simulink model "quadrator_model_v2"  (R2022b)
settings: Solver=FixedStepAuto  StartTime=0.0  StopTime=50  FixedStep=0.001  MaxStep=0.001  RelTol=1e-3
values from neighbouring files (symbols this model uses):
  l = readmatrix("RampTest_2023-06-05_114458")    [pwm2thrust_lut.m]
undefined symbols (not defined in the file or in its folder): manu
libraries: slpidlib x12, matrix_library x8, aerolibutil x7, sharedtransform x4, sharedutil x4, simulink_extras x3, shared6dof x1, aerolibasang x1, dspmathops x1
(part 1 of 2)
settings Model: Creator=ata  LastModifiedBy=ata
settings SolverCC: ZeroCrossAlgorithm=Adaptive
settings DataIOCC: Refine=4

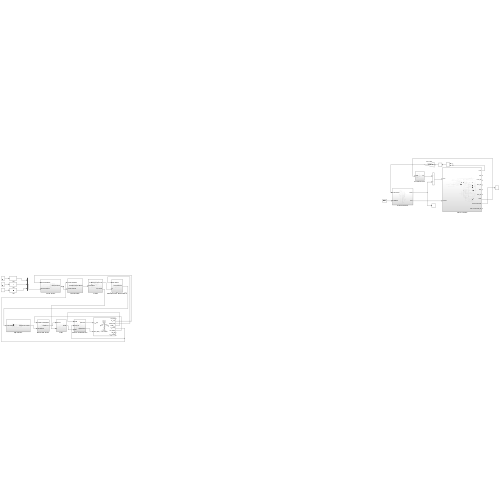
[thumbnail: Simulink's stored preview of the top-level diagram]
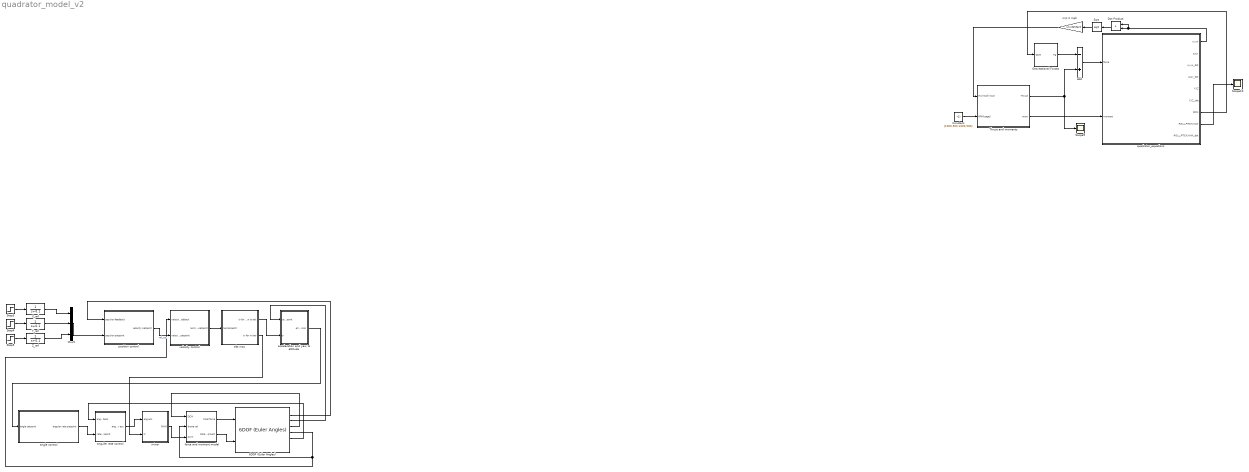
== system quadrator_model_v2 ==
  6DOF (Euler Angles) : shared6dof/6DOF (Euler Angles)  units=Metric (MKS)  mtype=Fixed  rep=Euler Angles  xme_0=[0 0 0]  Vm_0=[0.01 0.01 0.01]  eul_0=[0 0 0]  pm_0=[0 0 0]  mass_0=7.5  mass_e=0.5  mass_f=2.0  inertia=[0.3, 0,0 ; 0,0.3,0 ; 0,0, 0.2434]  inertia_e=eye(3)  inertia_f=2*eye(3)  k_quat=1.0  vre_flag=on  abi_flag=off  aMode=0  xme_statename=''  Vm_statename=''  eul_statename=''  quat_statename=''  pm_statename=''  mass_statename=''
  Add : Sum  Inputs=-+
  Constant : Constant  Value=[1000,500,1000,500]
  Dot Product : DotProduct  OutDataTypeStr=Inherit: Inherit via internal rule
  Gravitational Forces : Subsystem
  Mux5 : Mux  Inputs=3
  Scope10 : Scope
  Scope9 : Scope
  Sqrt : Sqrt
  Step3 : Step  After=2  SampleTime=0
  Step4 : Step  After=3  SampleTime=0
  Step5 : Step  After=-2  SampleTime=0
  Thrust and moments : Subsystem
  X_ref : TransferFcn  Denominator=[1 0.1]
  Y_ref : TransferFcn  Denominator=[1 0.1]
  Z_ref : TransferFcn  Denominator=[1 0.1]
  acceleration and yaw to attitude : Subsystem
  angle control : Subsystem
  anguler rate control : Subsystem
  force and moment model : Subsystem
  m/s 2 mph : Gain  Gain=1/2.23693629
  mixer : Subsystem
  position control : Subsystem
  quadrotor_equations : Subsystem
  tiltt max : Subsystem
  velocity control : Subsystem
  wires:
  quadrotor_equations/7(DCM) -> Gravitational Forces/1(DCM)
  Add/1 -> quadrotor_equations/1(force)
  quadrotor_equations/1(u,v,w) -> Dot Product/1, Dot Product/2
  Dot Product/1 -> Sqrt/1
  Constant/1 -> Thrust and moments/2(RPM(page))
  Sqrt/1 -> m/s 2 mph/1
  m/s 2 mph/1 -> Thrust and moments/1(Hız(mph)(row))
  Gravitational Forces/1(Fg) -> Add/1
  Thrust and moments/1(Thrust) -> Scope9/1, Add/2
  Thrust and moments/2(mom) -> quadrotor_equations/2(moment)
  quadrotor_equations/8(ROLL,PITCH,YAW) -> Scope10/1
  6DOF (Euler Angles)/2 -> position control/1(position feedback)
  6DOF (Euler Angles)/6 -> anguler rate control/1(angular rate feedback)
  6DOF (Euler Angles)/5 -> velocity control/1(velocity feedback), force and moment model/2(drone vel)
  6DOF (Euler Angles)/3 -> acceleration and yaw to attitude/1(yaw setpoint)
  position control/1(velocity setpoint) -> velocity control/2(velocity setpoint)  "vel_sp"
  velocity control/1(normalized thrust setpoint) -> tiltt max/1(nomalised tr)
  tiltt max/1(tr for Acc and Yaw to att) -> acceleration and yaw to attitude/2(tr)
  acceleration and yaw to attitude/1(error quaternion) -> angle control/1(angle setpoint)
  angle control/1(angular rate setpoint) -> anguler rate control/2(rate setpoint)
  anguler rate control/1(angular acc) -> mixer/1(ang acc)
  tiltt max/2(tr for mixer) -> mixer/2(tr)
  6DOF (Euler Angles)/4 -> force and moment model/1(DCM)
  mixer/1(PWM) -> force and moment model/3(pwm)
  force and moment model/1(total force) -> 6DOF (Euler Angles)/1
  force and moment model/2(total moment) -> 6DOF (Euler Angles)/2
  Mux5/1 -> position control/2(position setpoint)
  Y_ref/1 -> Mux5/2
  Step5/1 -> Z_ref/1
  Step3/1 -> X_ref/1
  X_ref/1 -> Mux5/1
  Z_ref/1 -> Mux5/3
  Step4/1 -> Y_ref/1

== system quadrator_model_v2/Gravitational Forces ==
  DCM : Inport
  G : Constant  Value=9.81
  Matrix Multiply : Product  Multiplication=Matrix(*)
  Product : Product
  Vector Concatenate : Concatenate  ConcatenateDimension=2
  mass : Constant  Value=7.5
  mass2 : Constant  Value=zeros(2,1)  VectorParams1D=off
  Fg : Outport
  wires:
  Matrix Multiply/1 -> Fg/1
  mass/1 -> Product/2
  mass2/1 -> Vector Concatenate/1
  G/1 -> Product/1
  Product/1 -> Vector Concatenate/2
  Vector Concatenate/1 -> Matrix Multiply/2
  DCM/1 -> Matrix Multiply/1

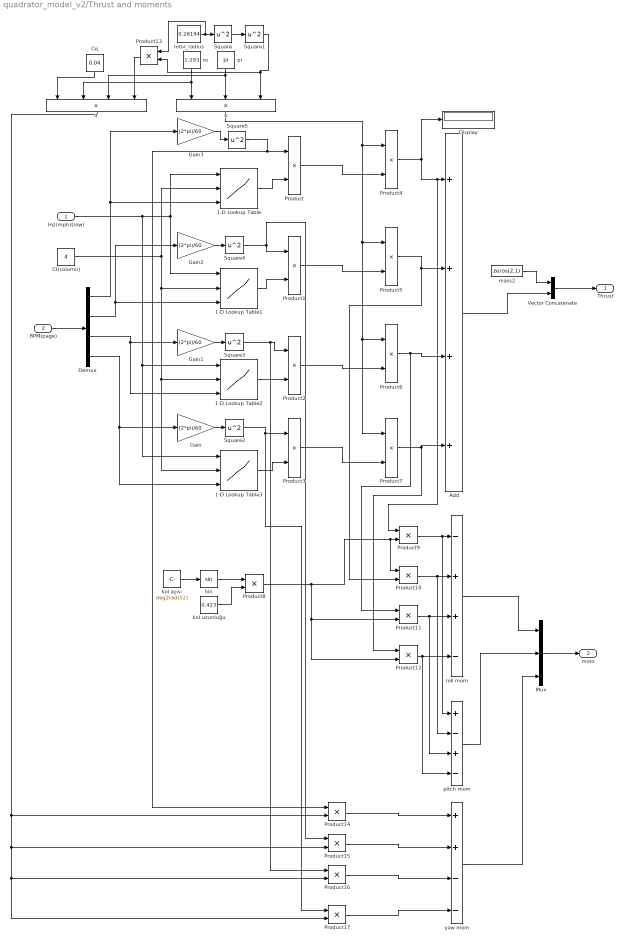
== system quadrator_model_v2/Thrust and moments ==
  Hız(mph)(row) : Inport
  RPM(page) : Inport  Port=2
  1-D Lookup Table : Lookup_n-D  NumberOfTableDimensions=3  BreakpointsForDimension1=manu(:,1)  BreakpointsForDimension2=(1:1:15)  BreakpointsForDimension3=(1000:1000:11000)  Table=manu  ExtrapMethod=Clip  UseLastTableValue=on  InternalRulePriority=Speed  RndMeth=Simplest
      settings: InputPortMap=u0,u1,u2
  1-D Lookup Table1 : Lookup_n-D  NumberOfTableDimensions=3  BreakpointsForDimension1=manu(:,1)  BreakpointsForDimension2=(1:1:15)  BreakpointsForDimension3=(1000:1000:11000)  Table=manu  ExtrapMethod=Clip  UseLastTableValue=on  InternalRulePriority=Speed  RndMeth=Simplest
      settings: InputPortMap=u0,u1,u2
  1-D Lookup Table2 : Lookup_n-D  NumberOfTableDimensions=3  BreakpointsForDimension1=manu(:,1)  BreakpointsForDimension2=(1:1:15)  BreakpointsForDimension3=(1000:1000:11000)  Table=manu  ExtrapMethod=Clip  UseLastTableValue=on  InternalRulePriority=Speed  RndMeth=Simplest
      settings: InputPortMap=u0,u1,u2
  1-D Lookup Table3 : Lookup_n-D  NumberOfTableDimensions=3  BreakpointsForDimension1=manu(:,1)  BreakpointsForDimension2=(1:1:15)  BreakpointsForDimension3=(1000:1000:11000)  Table=manu  ExtrapMethod=Clip  InternalRulePriority=Speed  RndMeth=Simplest
      settings: InputPortMap=u0,u1,u2
  Add : Sum  Inputs=++++
  Cq : Constant  Value=0.04
  Ct(column) : Constant  Value=4
  Demux : Demux
  Display : Display
  Gain{,1..3} (4 alike) : Gain  Gain=(2*pi)/60
  Mux : Mux  Inputs=3
  Product{,1..17} (18 alike) : Product
  Sin : Trigonometry
  Square{,1..5} (6 alike) : Math  Operator=square
  Vector Concatenate : Concatenate  ConcatenateDimension=2
  b : Product  Inputs=3
  d : Product  Inputs=4
  kol açısı : Constant  Value=deg2rad(52)
  kol uzunluğu : Constant  Value=0.423
  mass2 : Constant  Value=zeros(2,1)  VectorParams1D=off
  pi : Constant  Value=pi
  pitch mom : Sum  Inputs=+-+-
  ro : Constant  Value=1.293
  roll mom : Sum  Inputs=-++-
  rotor_radius : Constant  Value=0.28194
  yaw mom : Sum  Inputs=++--
  Thrust : Outport
  mom : Outport  Port=2
  wires:
  Product4/1 -> Display/1, Product9/1, Add/1
  Product7/1 -> Product12/1, Add/4
  Product2/1 -> Product6/2
  Square5/1 -> Product14/1, Product/1
  Product/1 -> Product4/2
  Gain2/1 -> Square4/1
  Product3/1 -> Product7/2
  Gain1/1 -> Square3/1
  Square3/1 -> Product2/1, Product16/1
  Square4/1 -> Product1/1, Product15/1
  1-D Lookup Table2/1 -> Product2/2
  Square2/1 -> Product17/1, Product3/1
  RPM(page)/1 -> Demux/1
  Gain3/1 -> Square5/1
  Product5/1 -> Product10/2, Add/2
  1-D Lookup Table/1 -> Product/2
  1-D Lookup Table3/1 -> Product3/2
  Gain/1 -> Square2/1
  1-D Lookup Table1/1 -> Product1/2
  pi/1 -> b/2, d/3
  Square1/1 -> Product13/2, b/3
  Product6/1 -> Product11/1, Add/3
  Demux/4 -> 1-D Lookup Table3/3, Gain/1
  ro/1 -> d/2, b/1
  Square/1 -> Square1/1
  Demux/1 -> Gain3/1, 1-D Lookup Table/3
  Demux/3 -> 1-D Lookup Table2/3, Gain1/1
  b/1 -> Product4/1, Product7/1, Product6/1, Product5/1
  Hız(mph)(row)/1 -> 1-D Lookup Table/1, 1-D Lookup Table1/1, 1-D Lookup Table3/1, 1-D Lookup Table2/1
  Demux/2 -> Gain2/1, 1-D Lookup Table1/3
  Ct(column)/1 -> 1-D Lookup Table/2, 1-D Lookup Table2/2, 1-D Lookup Table3/2, 1-D Lookup Table1/2
  rotor_radius/1 -> Product13/1, Square/1
  Product1/1 -> Product5/2
  mass2/1 -> Vector Concatenate/1
  Vector Concatenate/1 -> Thrust/1
  Add/1 -> Vector Concatenate/2
  kol açısı/1 -> Sin/1
  Sin/1 -> Product8/1
  kol uzunluğu/1 -> Product8/2
  Product8/1 -> Product12/2, Product11/2, Product10/1, Product9/2
  Product9/1 -> pitch mom/1, roll mom/1
  Product10/1 -> pitch mom/2, roll mom/2
  Product11/1 -> pitch mom/3, roll mom/3
  Product12/1 -> roll mom/4, pitch mom/4
  roll mom/1 -> Mux/1
  pitch mom/1 -> Mux/2
  Mux/1 -> mom/1
  Cq/1 -> d/1
  Product13/1 -> d/4
  yaw mom/1 -> Mux/3
  d/1 -> Product17/2, Product16/2, Product15/2, Product14/2
  Product14/1 -> yaw mom/1
  Product15/1 -> yaw mom/2
  Product16/1 -> yaw mom/3
  Product17/1 -> yaw mom/4

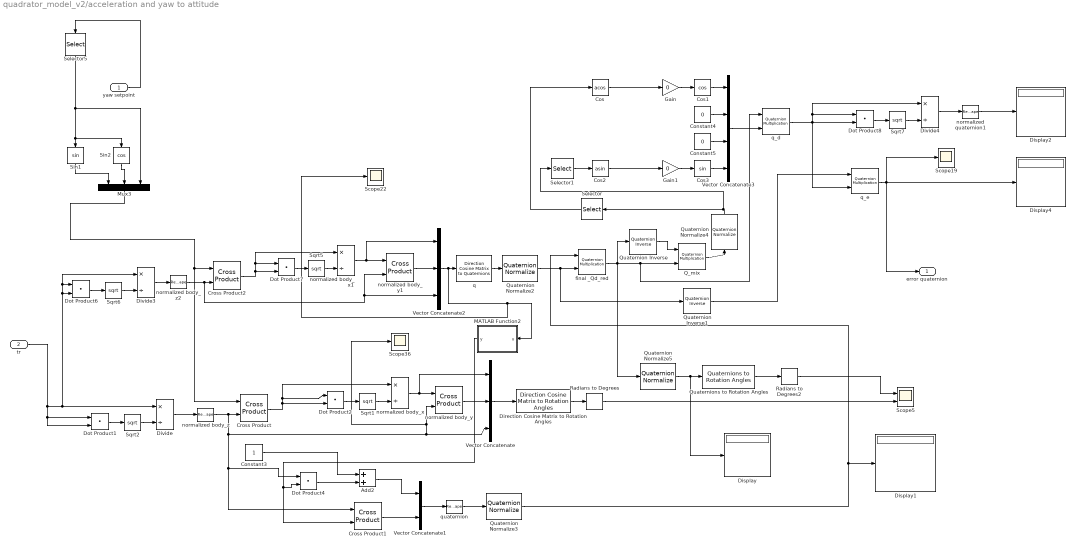
== system quadrator_model_v2/acceleration and yaw to attitude ==
  yaw setpoint : Inport
  tr : Inport  Port=2
  Add2 : Sum
  Constant3 : Constant
  Constant4 : Constant  Value=0
  Constant5 : Constant  Value=0
  Cos : Trigonometry  Operator=acos
  Cos1 : Trigonometry  Operator=cos
  Cos2 : Trigonometry  Operator=asin
  Cos3 : Trigonometry
  Cross Product : matrix_library/Cross Product
  Cross Product1 : matrix_library/Cross Product
  Cross Product2 : matrix_library/Cross Product
  Direction Cosine Matrix to Rotation Angles : sharedtransform/Direction Cosine Matrix to Rotation Angles  rotationOrder=ZYX  aMode=aMode  action=None  tolerance=eps(2)
      settings: LibrarySourceBlock=|
      | aerolibtransform2/Direction Cosine Matrix
      | to Rotation Angles
  Display{,1..2,4} (4 alike) : Display
  Divide : Product  Inputs=*/
  Divide3 : Product  Inputs=*/
  Divide4 : Product  Inputs=*/
  Dot Product{1..2,4,6..8} (6 alike) : DotProduct  OutDataTypeStr=Inherit: Inherit via internal rule
  Gain : Gain  Gain=0
  Gain1 : Gain  Gain=0
  MATLAB Function2 : MATLAB Function  TreatAsAtomicUnit=on
  Mux3 : Mux  Inputs=3
  Q_mix : aerolibutil/Quaternion Multiplication
  Quaternion Inverse : aerolibutil/Quaternion Inverse
  Quaternion Inverse1 : aerolibutil/Quaternion Inverse
  Quaternion Normalize{2..5} (4 alike) : sharedutil/Quaternion Normalize  aMode=aMode
  Quaternions to Rotation Angles : sharedtransform/Quaternions to Rotation Angles  rotationOrder=ZYX  aMode=aMode
  Radians to Degrees : simulink_extras/Transformations/Radians to Degrees
  Radians to Degrees2 : simulink_extras/Transformations/Radians to Degrees
  Scope19 : Scope
  Scope22 : Scope
  Scope36 : Scope
  Scope5 : Scope  NumInputPorts=2
  Selector : Selector  InputPortWidth=4  IndexOptions=Index vector (dialog)  Indices=[1]  OutputSizes=1
  Selector1 : Selector  InputPortWidth=4  IndexOptions=Index vector (dialog)  Indices=[4]  OutputSizes=1
  Selector5 : Selector  InputPortWidth=3  IndexOptions=Index vector (dialog)  Indices=[ 3]  OutputSizes=1
  Sin1 : Trigonometry
  Sin2 : Trigonometry  Operator=cos
  Sqrt{1..2,5..7} (5 alike) : Sqrt
  Vector Concatenate : Concatenate  NumInputs=3  Mode=Multidimensional array  ConcatenateDimension=2
  Vector Concatenate1 : Concatenate  ConcatenateDimension=2
  Vector Concatenate2 : Concatenate  NumInputs=3  Mode=Multidimensional array  ConcatenateDimension=2
  Vector Concatenate3 : Concatenate  NumInputs=4  Mode=Multidimensional array  ConcatenateDimension=2
  final _Qd_red : aerolibutil/Quaternion Multiplication
  normalized body_x : Product  Inputs=*/
  normalized body_x1 : Product  Inputs=*/
  normalized body_y : matrix_library/Cross Product
  normalized body_y1 : matrix_library/Cross Product
  normalized body_z : Reshape  OutputDimensionality=Column vector (2-D)
  normalized body_z2 : Reshape  OutputDimensionality=Column vector (2-D)
  normalized quaternion1 : Reshape  OutputDimensionality=Column vector (2-D)
  q : sharedtransform/Direction Cosine Matrix  to Quaternions  aMode=0  action=None  tolerance=eps(2)
      settings: LibrarySourceBlock=|
      | aerolibtransform2/Direction Cosine Matrix
      | to Quaternions
  q_d : aerolibutil/Quaternion Multiplication
  q_e : aerolibutil/Quaternion Multiplication
  quaternion : Reshape  OutputDimensionality=Row vector (2-D)
  error quaternion : Outport
  wires:
  yaw setpoint/1 -> Selector5/1
  Cos/1 -> Gain/1
  q/1 -> Quaternion Normalize2/1
  Divide4/1 -> normalized quaternion1/1
  Cos3/1 -> Vector Concatenate3/4
  Selector1/1 -> Cos2/1
  Add2/1 -> Vector Concatenate1/1
  Quaternion Inverse/1 -> Q_mix/1
  Cross Product1/1 -> Vector Concatenate1/2
  Vector Concatenate/1 -> Direction Cosine Matrix to Rotation Angles/1
  Sqrt1/1 -> normalized body_x/2
  Dot Product7/1 -> Sqrt5/1
  Sin1/1 -> Mux3/1
  Radians to Degrees/1 -> Scope5/2
  q_d/1 -> Divide4/1, Dot Product8/1, Dot Product8/2, q_e/2
  Quaternion Normalize3/1 -> Display1/1, final _Qd_red/1
  final _Qd_red/1 -> Quaternion Normalize5/1, Quaternion Inverse/1, q_d/1, Q_mix/2
  Radians to Degrees2/1 -> Scope5/1
  Sqrt2/1 -> Divide/2
  normalized body_x1/1 -> normalized body_y1/1, Vector Concatenate2/1
  Sqrt6/1 -> Divide3/2
  Quaternion Normalize5/1 -> Display/1, Quaternions to Rotation Angles/1
  Sqrt5/1 -> normalized body_x1/2
  Cos1/1 -> Vector Concatenate3/1
  Constant5/1 -> Vector Concatenate3/3
  Gain/1 -> Cos1/1
  Cos2/1 -> Gain1/1
  Divide/1 -> normalized body_z/1
  Quaternion Normalize4/1 -> Selector1/1, Selector/1
  Selector/1 -> Cos/1
  Gain1/1 -> Cos3/1
  normalized body_z/1 -> Cross Product1/1, Dot Product4/1, Scope36/1, normalized body_y/2, Vector Concatenate/3, Cross Product/2
  Dot Product1/1 -> Sqrt2/1
  Quaternions to Rotation Angles/1 -> Radians to Degrees2/1
  Quaternion Inverse1/1 -> q_e/1
  Dot Product2/1 -> Sqrt1/1
  Sin2/1 -> Mux3/2
  Cross Product/1 -> normalized body_x/1, Dot Product2/1, Dot Product2/2
  normalized body_x/1 -> Vector Concatenate/1, normalized body_y/1
  Quaternion Normalize2/1 -> final _Qd_red/2, Quaternion Inverse1/1
  Vector Concatenate1/1 -> quaternion/1
  Vector Concatenate3/1 -> q_d/2
  Direction Cosine Matrix to Rotation Angles/1 -> Radians to Degrees/1
  normalized body_z2/1 -> Cross Product2/2, Vector Concatenate2/3, normalized body_y1/2
  Constant4/1 -> Vector Concatenate3/2
  tr/1 -> Divide/1, Dot Product6/2, Divide3/1, Dot Product6/1, Dot Product1/2, Dot Product1/1
  quaternion/1 -> Quaternion Normalize3/1
  Selector5/1 -> Mux3/3, Sin2/1, Sin1/1
  Dot Product8/1 -> Sqrt7/1
  Sqrt7/1 -> Divide4/2
  q_e/1 -> error quaternion/1, Scope19/1, Display4/1
  Dot Product6/1 -> Sqrt6/1
  Dot Product4/1 -> Add2/2
  normalized body_y/1 -> Vector Concatenate/2
  Divide3/1 -> normalized body_z2/1
  normalized quaternion1/1 -> Display2/1
  Q_mix/1 -> Quaternion Normalize4/1
  Mux3/1 -> Cross Product2/1, Cross Product/1
  normalized body_y1/1 -> Vector Concatenate2/2
  MATLAB Function2/1(y) -> Cross Product1/2, Dot Product4/2
  Vector Concatenate2/1 -> q/1, Scope22/1, MATLAB Function2/1(u)
  Constant3/1 -> Add2/1
  Cross Product2/1 -> normalized body_x1/1, Dot Product7/1, Dot Product7/2

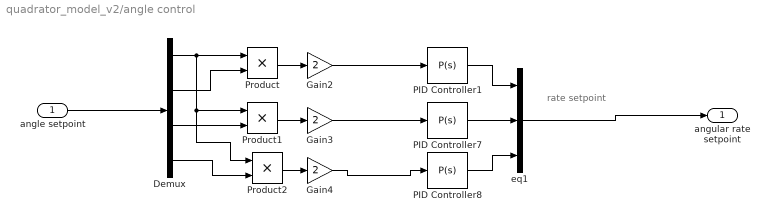
== system quadrator_model_v2/angle control ==
  note: rate setpoint
  angle setpoint : Inport
  Demux : Demux
  Gain2 : Gain  Gain=2
  Gain3 : Gain  Gain=2
  Gain4 : Gain  Gain=2
  PID Controller1 : slpidlib/PID Controller  Controller=P  Form=Parallel  TimeDomain=Continuous-time  UseExternalTs=off  SampleTime=-1  IntegratorMethod=Forward Euler  FilterMethod=Forward Euler  ControllerParametersSource=internal  P=20  I=9.5219837376893e-06  UseKiTs=off  D=-1.0490403925014e-05  N=1.72044274974478  UseFilter=on  TunerSelectOption=Transfer Function Based (PID Tuner App)  InitialConditionSource=internal  InitialConditionForIntegrator=0  InitialConditionForFilter=0  DifferentiatorICPrevScaledInput=0  ExternalReset=none  TrackingMode=off  Kt=1  LimitOutput=off  SatLimitsSource=internal  UpperSaturationLimit=inf  LowerSaturationLimit=-inf  LinearizeAsGain=on  AntiWindupMode=none  Kb=1  LimitIntegrator=off  UpperIntegratorSaturationLimit=inf  LowerIntegratorSaturationLimit=-inf  POutMin=[]  POutMax=[]  IOutMin=[]  IOutMax=[]  DOutMin=[]  DOutMax=[]  NOutMin=[]  NOutMax=[]  SumOutMin=[]  SumOutMax=[]  SaturationOutMin=[]  SaturationOutMax=[]  PParamMin=[]  PParamMax=[]  IParamMin=[]  IParamMax=[]  DParamMin=[]  DParamMax=[]  NParamMin=[]  NParamMax=[]  KbParamMin=[]  KbParamMax=[]  KtParamMin=[]  KtParamMax=[]  KbOutMin=[]  KbOutMax=[]  KtOutMin=[]  KtOutMax=[]  IntegratorOutMin=[]  IntegratorOutMax=[]  FilterOutMin=[]  FilterOutMax=[]  SumI1OutMin=[]  SumI1OutMax=[]  SumI2OutMin=[]  SumI2OutMax=[]  SumI3OutMin=[]  SumI3OutMax=[]  SumI4OutMin=[]  SumI4OutMax=[]  SumDOutMin=[]  SumDOutMax=[]  DifferentiatorOutMin=[]  DifferentiatorOutMax=[]  FilterDiffOutCoefMin=[]  FilterDiffOutCoefMax=[]  ReciprocalOutMin=[]  ReciprocalOutMax=[]  SumDenOutMin=[]  SumDenOutMax=[]  SumNumOutMin=[]  SumNumOutMax=[]  DivideOutMin=[]  DivideOutMax=[]  UdiffTsProdOutMin=[]  UdiffTsProdOutMax=[]  NTsProdOutMin=[]  NTsProdOutMax=[]  UintegralTsProdOutMin=[]  UintegralTsProdOutMax=[]  UngainTsProdOutMin=[]  UngainTsProdOutMax=[]  ClampingZeroOutDataTypeStr=Inherit: Inherit via back propagation  ClampingZeroOutMin=[]  ClampingZeroOutMax=[]  FilterDenConstantOutDataTypeStr=Inherit: Inherit via back propagation  FilterDenConstantOutMin=[]  FilterDenConstantOutMax=[]  PCopyOutDataTypeStr=Inherit: Inherit via back propagation  PCopyOutMin=[]  PCopyOutMax=[]  NCopyOutDataTypeStr=Inherit: Inherit via back propagation  NCopyOutMin=[]  NCopyOutMax=[]  IntegratorContinuousStateAttributes=''  IntegratorStateMustResolveToSignalObject=off  IntegratorRTWStateStorageClass=Auto  FilterContinuousStateAttributes=''  FilterStateMustResolveToSignalObject=off  FilterRTWStateStorageClass=Auto  ParallelPVariant=InternalParameters  IdealPVariant=Disabled  IVariant=Disabled  DVariant=Disabled  IntegratorVariant=Disabled  SatVariant=Disabled  AWVariant=Disabled  PCopyVariant=Disabled  TRVariant=Disabled  FdbkBlocksVariant=Forward  IdealPFdbkVariant=Disabled  SatFdbkVariant=Disabled  DerivativeFilterVariant=Disabled  NVariant=Disabled  NCopyVariant=Disabled_SignalSpec  FilterICVariant=Disabled  IntegratorICVariant=Disabled  ExternalResetVariant=Disabled  TRSumVariant=Passthrough  SumFdbkVariant=Disabled  SumVariant=Passthrough_P  TsampFilterVariant=InternalTs  TsampNgainVariant=Passthrough  TsampIntegralVariant=Disabled_SignalSpec  ExternalSaturationOutDataTypeStr=Inherit: Same as second input
  PID Controller7 : slpidlib/PID Controller  Controller=P  Form=Parallel  TimeDomain=Continuous-time  UseExternalTs=off  SampleTime=-1  IntegratorMethod=Forward Euler  FilterMethod=Forward Euler  ControllerParametersSource=internal  P=9.5  I=-6.49908455563329e-05  UseKiTs=off  D=-0.683044885728483  N=43.2582215401561  UseFilter=on  TunerSelectOption=Transfer Function Based (PID Tuner App)  InitialConditionSource=internal  InitialConditionForIntegrator=0  InitialConditionForFilter=0  DifferentiatorICPrevScaledInput=0  ExternalReset=none  TrackingMode=off  Kt=1  LimitOutput=off  SatLimitsSource=internal  UpperSaturationLimit=inf  LowerSaturationLimit=-inf  LinearizeAsGain=on  AntiWindupMode=none  Kb=1  LimitIntegrator=off  UpperIntegratorSaturationLimit=inf  LowerIntegratorSaturationLimit=-inf  POutMin=[]  POutMax=[]  IOutMin=[]  IOutMax=[]  DOutMin=[]  DOutMax=[]  NOutMin=[]  NOutMax=[]  SumOutMin=[]  SumOutMax=[]  SaturationOutMin=[]  SaturationOutMax=[]  PParamMin=[]  PParamMax=[]  IParamMin=[]  IParamMax=[]  DParamMin=[]  DParamMax=[]  NParamMin=[]  NParamMax=[]  KbParamMin=[]  KbParamMax=[]  KtParamMin=[]  KtParamMax=[]  KbOutMin=[]  KbOutMax=[]  KtOutMin=[]  KtOutMax=[]  IntegratorOutMin=[]  IntegratorOutMax=[]  FilterOutMin=[]  FilterOutMax=[]  SumI1OutMin=[]  SumI1OutMax=[]  SumI2OutMin=[]  SumI2OutMax=[]  SumI3OutMin=[]  SumI3OutMax=[]  SumI4OutMin=[]  SumI4OutMax=[]  SumDOutMin=[]  SumDOutMax=[]  DifferentiatorOutMin=[]  DifferentiatorOutMax=[]  FilterDiffOutCoefMin=[]  FilterDiffOutCoefMax=[]  ReciprocalOutMin=[]  ReciprocalOutMax=[]  SumDenOutMin=[]  SumDenOutMax=[]  SumNumOutMin=[]  SumNumOutMax=[]  DivideOutMin=[]  DivideOutMax=[]  UdiffTsProdOutMin=[]  UdiffTsProdOutMax=[]  NTsProdOutMin=[]  NTsProdOutMax=[]  UintegralTsProdOutMin=[]  UintegralTsProdOutMax=[]  UngainTsProdOutMin=[]  UngainTsProdOutMax=[]  ClampingZeroOutDataTypeStr=Inherit: Inherit via back propagation  ClampingZeroOutMin=[]  ClampingZeroOutMax=[]  FilterDenConstantOutDataTypeStr=Inherit: Inherit via back propagation  FilterDenConstantOutMin=[]  FilterDenConstantOutMax=[]  PCopyOutDataTypeStr=Inherit: Inherit via back propagation  PCopyOutMin=[]  PCopyOutMax=[]  NCopyOutDataTypeStr=Inherit: Inherit via back propagation  NCopyOutMin=[]  NCopyOutMax=[]  IntegratorContinuousStateAttributes=''  IntegratorStateMustResolveToSignalObject=off  IntegratorRTWStateStorageClass=Auto  FilterContinuousStateAttributes=''  FilterStateMustResolveToSignalObject=off  FilterRTWStateStorageClass=Auto  ParallelPVariant=InternalParameters  IdealPVariant=Disabled  IVariant=Disabled  DVariant=Disabled  IntegratorVariant=Disabled  SatVariant=Disabled  AWVariant=Disabled  PCopyVariant=Disabled  TRVariant=Disabled  FdbkBlocksVariant=Forward  IdealPFdbkVariant=Disabled  SatFdbkVariant=Disabled  DerivativeFilterVariant=Disabled  NVariant=Disabled  NCopyVariant=Disabled_SignalSpec  FilterICVariant=Disabled  IntegratorICVariant=Disabled  ExternalResetVariant=Disabled  TRSumVariant=Passthrough  SumFdbkVariant=Disabled  SumVariant=Passthrough_P  TsampFilterVariant=InternalTs  TsampNgainVariant=Passthrough  TsampIntegralVariant=Disabled_SignalSpec  ExternalSaturationOutDataTypeStr=Inherit: Same as second input
  PID Controller8 : slpidlib/PID Controller  Controller=P  Form=Parallel  TimeDomain=Continuous-time  UseExternalTs=off  SampleTime=-1  IntegratorMethod=Forward Euler  FilterMethod=Forward Euler  ControllerParametersSource=internal  P=6.5  I=9.5219837376893e-06  UseKiTs=off  D=-1.0490403925014e-05  N=1.72044274974478  UseFilter=on  TunerSelectOption=Transfer Function Based (PID Tuner App)  InitialConditionSource=internal  InitialConditionForIntegrator=0  InitialConditionForFilter=0  DifferentiatorICPrevScaledInput=0  ExternalReset=none  TrackingMode=off  Kt=1  LimitOutput=off  SatLimitsSource=internal  UpperSaturationLimit=inf  LowerSaturationLimit=-inf  LinearizeAsGain=on  AntiWindupMode=none  Kb=1  LimitIntegrator=off  UpperIntegratorSaturationLimit=inf  LowerIntegratorSaturationLimit=-inf  POutMin=[]  POutMax=[]  IOutMin=[]  IOutMax=[]  DOutMin=[]  DOutMax=[]  NOutMin=[]  NOutMax=[]  SumOutMin=[]  SumOutMax=[]  SaturationOutMin=[]  SaturationOutMax=[]  PParamMin=[]  PParamMax=[]  IParamMin=[]  IParamMax=[]  DParamMin=[]  DParamMax=[]  NParamMin=[]  NParamMax=[]  KbParamMin=[]  KbParamMax=[]  KtParamMin=[]  KtParamMax=[]  KbOutMin=[]  KbOutMax=[]  KtOutMin=[]  KtOutMax=[]  IntegratorOutMin=[]  IntegratorOutMax=[]  FilterOutMin=[]  FilterOutMax=[]  SumI1OutMin=[]  SumI1OutMax=[]  SumI2OutMin=[]  SumI2OutMax=[]  SumI3OutMin=[]  SumI3OutMax=[]  SumI4OutMin=[]  SumI4OutMax=[]  SumDOutMin=[]  SumDOutMax=[]  DifferentiatorOutMin=[]  DifferentiatorOutMax=[]  FilterDiffOutCoefMin=[]  FilterDiffOutCoefMax=[]  ReciprocalOutMin=[]  ReciprocalOutMax=[]  SumDenOutMin=[]  SumDenOutMax=[]  SumNumOutMin=[]  SumNumOutMax=[]  DivideOutMin=[]  DivideOutMax=[]  UdiffTsProdOutMin=[]  UdiffTsProdOutMax=[]  NTsProdOutMin=[]  NTsProdOutMax=[]  UintegralTsProdOutMin=[]  UintegralTsProdOutMax=[]  UngainTsProdOutMin=[]  UngainTsProdOutMax=[]  ClampingZeroOutDataTypeStr=Inherit: Inherit via back propagation  ClampingZeroOutMin=[]  ClampingZeroOutMax=[]  FilterDenConstantOutDataTypeStr=Inherit: Inherit via back propagation  FilterDenConstantOutMin=[]  FilterDenConstantOutMax=[]  PCopyOutDataTypeStr=Inherit: Inherit via back propagation  PCopyOutMin=[]  PCopyOutMax=[]  NCopyOutDataTypeStr=Inherit: Inherit via back propagation  NCopyOutMin=[]  NCopyOutMax=[]  IntegratorContinuousStateAttributes=''  IntegratorStateMustResolveToSignalObject=off  IntegratorRTWStateStorageClass=Auto  FilterContinuousStateAttributes=''  FilterStateMustResolveToSignalObject=off  FilterRTWStateStorageClass=Auto  ParallelPVariant=InternalParameters  IdealPVariant=Disabled  IVariant=Disabled  DVariant=Disabled  IntegratorVariant=Disabled  SatVariant=Disabled  AWVariant=Disabled  PCopyVariant=Disabled  TRVariant=Disabled  FdbkBlocksVariant=Forward  IdealPFdbkVariant=Disabled  SatFdbkVariant=Disabled  DerivativeFilterVariant=Disabled  NVariant=Disabled  NCopyVariant=Disabled_SignalSpec  FilterICVariant=Disabled  IntegratorICVariant=Disabled  ExternalResetVariant=Disabled  TRSumVariant=Passthrough  SumFdbkVariant=Disabled  SumVariant=Passthrough_P  TsampFilterVariant=InternalTs  TsampNgainVariant=Passthrough  TsampIntegralVariant=Disabled_SignalSpec  ExternalSaturationOutDataTypeStr=Inherit: Same as second input
  Product : Product
  Product1 : Product
  Product2 : Product
  eq1 : Mux  Inputs=3
  angular rate setpoint : Outport
  wires:
  angle setpoint/1 -> Demux/1
  Gain3/1 -> PID Controller7/1
  Gain4/1 -> PID Controller8/1
  eq1/1 -> angular rate setpoint/1
  Product/1 -> Gain2/1
  Product1/1 -> Gain3/1
  Gain2/1 -> PID Controller1/1
  PID Controller8/1 -> eq1/3
  Demux/2 -> Product/2
  PID Controller1/1 -> eq1/1
  Product2/1 -> Gain4/1
  Demux/4 -> Product2/2
  Demux/3 -> Product1/2
  Demux/1 -> Product2/1, Product1/1, Product/1
  PID Controller7/1 -> eq1/2

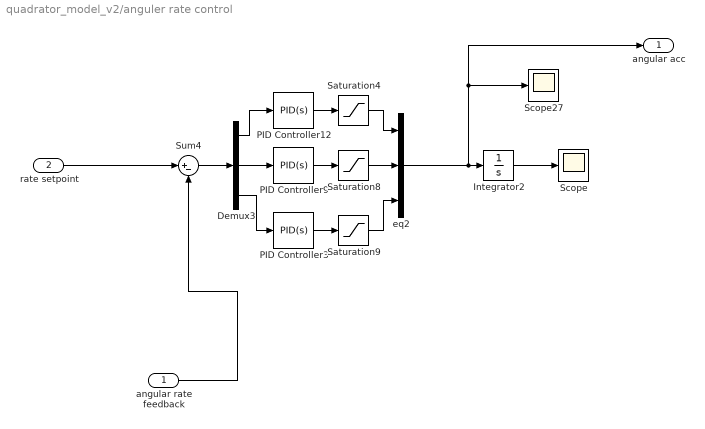
== system quadrator_model_v2/anguler rate control ==
  angular rate feedback : Inport
  rate setpoint : Inport  Port=2
  Demux3 : Demux  Outputs=3
  Integrator2 : Integrator
  PID Controller12 : slpidlib/PID Controller  Controller=PID  Form=Parallel  TimeDomain=Continuous-time  UseExternalTs=off  SampleTime=-1  IntegratorMethod=Forward Euler  FilterMethod=Forward Euler  ControllerParametersSource=internal  P=0.0462030393294061  I=0.000816085221651918  UseKiTs=off  D=8.77448123465224e-06  N=36.46824066771  UseFilter=on  TunerSelectOption=Transfer Function Based (PID Tuner App)  InitialConditionSource=internal  InitialConditionForIntegrator=0  InitialConditionForFilter=0  DifferentiatorICPrevScaledInput=0  ExternalReset=none  TrackingMode=off  Kt=1  LimitOutput=off  SatLimitsSource=internal  UpperSaturationLimit=inf  LowerSaturationLimit=-inf  LinearizeAsGain=on  AntiWindupMode=none  Kb=1  LimitIntegrator=off  UpperIntegratorSaturationLimit=inf  LowerIntegratorSaturationLimit=-inf  POutMin=[]  POutMax=[]  IOutMin=[]  IOutMax=[]  DOutMin=[]  DOutMax=[]  NOutMin=[]  NOutMax=[]  SumOutMin=[]  SumOutMax=[]  SaturationOutMin=[]  SaturationOutMax=[]  PParamMin=[]  PParamMax=[]  IParamMin=[]  IParamMax=[]  DParamMin=[]  DParamMax=[]  NParamMin=[]  NParamMax=[]  KbParamMin=[]  KbParamMax=[]  KtParamMin=[]  KtParamMax=[]  KbOutMin=[]  KbOutMax=[]  KtOutMin=[]  KtOutMax=[]  IntegratorOutMin=[]  IntegratorOutMax=[]  FilterOutMin=[]  FilterOutMax=[]  SumI1OutMin=[]  SumI1OutMax=[]  SumI2OutMin=[]  SumI2OutMax=[]  SumI3OutMin=[]  SumI3OutMax=[]  SumI4OutMin=[]  SumI4OutMax=[]  SumDOutMin=[]  SumDOutMax=[]  DifferentiatorOutMin=[]  DifferentiatorOutMax=[]  FilterDiffOutCoefMin=[]  FilterDiffOutCoefMax=[]  ReciprocalOutMin=[]  ReciprocalOutMax=[]  SumDenOutMin=[]  SumDenOutMax=[]  SumNumOutMin=[]  SumNumOutMax=[]  DivideOutMin=[]  DivideOutMax=[]  UdiffTsProdOutMin=[]  UdiffTsProdOutMax=[]  NTsProdOutMin=[]  NTsProdOutMax=[]  UintegralTsProdOutMin=[]  UintegralTsProdOutMax=[]  UngainTsProdOutMin=[]  UngainTsProdOutMax=[]  ClampingZeroOutDataTypeStr=Inherit: Inherit via back propagation  ClampingZeroOutMin=[]  ClampingZeroOutMax=[]  FilterDenConstantOutDataTypeStr=Inherit: Inherit via back propagation  FilterDenConstantOutMin=[]  FilterDenConstantOutMax=[]  PCopyOutDataTypeStr=Inherit: Inherit via back propagation  PCopyOutMin=[]  PCopyOutMax=[]  NCopyOutDataTypeStr=Inherit: Inherit via back propagation  NCopyOutMin=[]  NCopyOutMax=[]  IntegratorContinuousStateAttributes=''  IntegratorStateMustResolveToSignalObject=off  IntegratorRTWStateStorageClass=Auto  FilterContinuousStateAttributes=''  FilterStateMustResolveToSignalObject=off  FilterRTWStateStorageClass=Auto  ParallelPVariant=InternalParameters  IdealPVariant=Disabled  IVariant=InternalParameters  DVariant=InternalParameters  IntegratorVariant=Continuous  SatVariant=Disabled  AWVariant=Passthrough  PCopyVariant=Disabled  TRVariant=Disabled  FdbkBlocksVariant=Forward  IdealPFdbkVariant=Disabled  SatFdbkVariant=Disabled  DerivativeFilterVariant=ContFilter  NVariant=InternalParameters  NCopyVariant=Disabled  FilterICVariant=InternalICsFilter  IntegratorICVariant=InternalICs  ExternalResetVariant=Disabled  TRSumVariant=Passthrough  SumFdbkVariant=Disabled  SumVariant=Sum_PID  TsampFilterVariant=InternalTs  TsampNgainVariant=Passthrough  TsampIntegralVariant=Passthrough  ExternalSaturationOutDataTypeStr=Inherit: Same as second input
  PID Controller3 : slpidlib/PID Controller  Controller=PID  Form=Parallel  TimeDomain=Continuous-time  UseExternalTs=off  SampleTime=-1  IntegratorMethod=Forward Euler  FilterMethod=Forward Euler  ControllerParametersSource=internal  P=0.0108449415865821  I=0.0207444576872011  UseKiTs=off  D=-0.000228542440670992  N=17.2044274974478  UseFilter=on  TunerSelectOption=Transfer Function Based (PID Tuner App)  InitialConditionSource=internal  InitialConditionForIntegrator=0  InitialConditionForFilter=0  DifferentiatorICPrevScaledInput=0  ExternalReset=none  TrackingMode=off  Kt=1  LimitOutput=off  SatLimitsSource=internal  UpperSaturationLimit=inf  LowerSaturationLimit=-inf  LinearizeAsGain=on  AntiWindupMode=none  Kb=1  LimitIntegrator=off  UpperIntegratorSaturationLimit=inf  LowerIntegratorSaturationLimit=-inf  POutMin=[]  POutMax=[]  IOutMin=[]  IOutMax=[]  DOutMin=[]  DOutMax=[]  NOutMin=[]  NOutMax=[]  SumOutMin=[]  SumOutMax=[]  SaturationOutMin=[]  SaturationOutMax=[]  PParamMin=[]  PParamMax=[]  IParamMin=[]  IParamMax=[]  DParamMin=[]  DParamMax=[]  NParamMin=[]  NParamMax=[]  KbParamMin=[]  KbParamMax=[]  KtParamMin=[]  KtParamMax=[]  KbOutMin=[]  KbOutMax=[]  KtOutMin=[]  KtOutMax=[]  IntegratorOutMin=[]  IntegratorOutMax=[]  FilterOutMin=[]  FilterOutMax=[]  SumI1OutMin=[]  SumI1OutMax=[]  SumI2OutMin=[]  SumI2OutMax=[]  SumI3OutMin=[]  SumI3OutMax=[]  SumI4OutMin=[]  SumI4OutMax=[]  SumDOutMin=[]  SumDOutMax=[]  DifferentiatorOutMin=[]  DifferentiatorOutMax=[]  FilterDiffOutCoefMin=[]  FilterDiffOutCoefMax=[]  ReciprocalOutMin=[]  ReciprocalOutMax=[]  SumDenOutMin=[]  SumDenOutMax=[]  SumNumOutMin=[]  SumNumOutMax=[]  DivideOutMin=[]  DivideOutMax=[]  UdiffTsProdOutMin=[]  UdiffTsProdOutMax=[]  NTsProdOutMin=[]  NTsProdOutMax=[]  UintegralTsProdOutMin=[]  UintegralTsProdOutMax=[]  UngainTsProdOutMin=[]  UngainTsProdOutMax=[]  ClampingZeroOutDataTypeStr=Inherit: Inherit via back propagation  ClampingZeroOutMin=[]  ClampingZeroOutMax=[]  FilterDenConstantOutDataTypeStr=Inherit: Inherit via back propagation  FilterDenConstantOutMin=[]  FilterDenConstantOutMax=[]  PCopyOutDataTypeStr=Inherit: Inherit via back propagation  PCopyOutMin=[]  PCopyOutMax=[]  NCopyOutDataTypeStr=Inherit: Inherit via back propagation  NCopyOutMin=[]  NCopyOutMax=[]  IntegratorContinuousStateAttributes=''  IntegratorStateMustResolveToSignalObject=off  IntegratorRTWStateStorageClass=Auto  FilterContinuousStateAttributes=''  FilterStateMustResolveToSignalObject=off  FilterRTWStateStorageClass=Auto  ParallelPVariant=InternalParameters  IdealPVariant=Disabled  IVariant=InternalParameters  DVariant=InternalParameters  IntegratorVariant=Continuous  SatVariant=Disabled  AWVariant=Passthrough  PCopyVariant=Disabled  TRVariant=Disabled  FdbkBlocksVariant=Forward  IdealPFdbkVariant=Disabled  SatFdbkVariant=Disabled  DerivativeFilterVariant=ContFilter  NVariant=InternalParameters  NCopyVariant=Disabled  FilterICVariant=InternalICsFilter  IntegratorICVariant=InternalICs  ExternalResetVariant=Disabled  TRSumVariant=Passthrough  SumFdbkVariant=Disabled  SumVariant=Sum_PID  TsampFilterVariant=InternalTs  TsampNgainVariant=Passthrough  TsampIntegralVariant=Passthrough  ExternalSaturationOutDataTypeStr=Inherit: Same as second input
  PID Controller9 : slpidlib/PID Controller  Controller=PID  Form=Parallel  TimeDomain=Continuous-time  UseExternalTs=off  SampleTime=-1  IntegratorMethod=Forward Euler  FilterMethod=Forward Euler  ControllerParametersSource=internal  P=0.0729107873230942  I=0.00139465457742601  UseKiTs=off  D=-1.53649599244316e-05  N=17.2044274974478  UseFilter=on  TunerSelectOption=Transfer Function Based (PID Tuner App)  InitialConditionSource=internal  InitialConditionForIntegrator=0  InitialConditionForFilter=0  DifferentiatorICPrevScaledInput=0  ExternalReset=none  TrackingMode=off  Kt=1  LimitOutput=off  SatLimitsSource=internal  UpperSaturationLimit=inf  LowerSaturationLimit=-inf  LinearizeAsGain=on  AntiWindupMode=none  Kb=1  LimitIntegrator=off  UpperIntegratorSaturationLimit=inf  LowerIntegratorSaturationLimit=-inf  POutMin=[]  POutMax=[]  IOutMin=[]  IOutMax=[]  DOutMin=[]  DOutMax=[]  NOutMin=[]  NOutMax=[]  SumOutMin=[]  SumOutMax=[]  SaturationOutMin=[]  SaturationOutMax=[]  PParamMin=[]  PParamMax=[]  IParamMin=[]  IParamMax=[]  DParamMin=[]  DParamMax=[]  NParamMin=[]  NParamMax=[]  KbParamMin=[]  KbParamMax=[]  KtParamMin=[]  KtParamMax=[]  KbOutMin=[]  KbOutMax=[]  KtOutMin=[]  KtOutMax=[]  IntegratorOutMin=[]  IntegratorOutMax=[]  FilterOutMin=[]  FilterOutMax=[]  SumI1OutMin=[]  SumI1OutMax=[]  SumI2OutMin=[]  SumI2OutMax=[]  SumI3OutMin=[]  SumI3OutMax=[]  SumI4OutMin=[]  SumI4OutMax=[]  SumDOutMin=[]  SumDOutMax=[]  DifferentiatorOutMin=[]  DifferentiatorOutMax=[]  FilterDiffOutCoefMin=[]  FilterDiffOutCoefMax=[]  ReciprocalOutMin=[]  ReciprocalOutMax=[]  SumDenOutMin=[]  SumDenOutMax=[]  SumNumOutMin=[]  SumNumOutMax=[]  DivideOutMin=[]  DivideOutMax=[]  UdiffTsProdOutMin=[]  UdiffTsProdOutMax=[]  NTsProdOutMin=[]  NTsProdOutMax=[]  UintegralTsProdOutMin=[]  UintegralTsProdOutMax=[]  UngainTsProdOutMin=[]  UngainTsProdOutMax=[]  ClampingZeroOutDataTypeStr=Inherit: Inherit via back propagation  ClampingZeroOutMin=[]  ClampingZeroOutMax=[]  FilterDenConstantOutDataTypeStr=Inherit: Inherit via back propagation  FilterDenConstantOutMin=[]  FilterDenConstantOutMax=[]  PCopyOutDataTypeStr=Inherit: Inherit via back propagation  PCopyOutMin=[]  PCopyOutMax=[]  NCopyOutDataTypeStr=Inherit: Inherit via back propagation  NCopyOutMin=[]  NCopyOutMax=[]  IntegratorContinuousStateAttributes=''  IntegratorStateMustResolveToSignalObject=off  IntegratorRTWStateStorageClass=Auto  FilterContinuousStateAttributes=''  FilterStateMustResolveToSignalObject=off  FilterRTWStateStorageClass=Auto  ParallelPVariant=InternalParameters  IdealPVariant=Disabled  IVariant=InternalParameters  DVariant=InternalParameters  IntegratorVariant=Continuous  SatVariant=Disabled  AWVariant=Passthrough  PCopyVariant=Disabled  TRVariant=Disabled  FdbkBlocksVariant=Forward  IdealPFdbkVariant=Disabled  SatFdbkVariant=Disabled  DerivativeFilterVariant=ContFilter  NVariant=InternalParameters  NCopyVariant=Disabled  FilterICVariant=InternalICsFilter  IntegratorICVariant=InternalICs  ExternalResetVariant=Disabled  TRSumVariant=Passthrough  SumFdbkVariant=Disabled  SumVariant=Sum_PID  TsampFilterVariant=InternalTs  TsampNgainVariant=Passthrough  TsampIntegralVariant=Passthrough  ExternalSaturationOutDataTypeStr=Inherit: Same as second input
  Saturation4 : Saturate  UpperLimit=1.047*5  LowerLimit=-0.5*5
  Saturation8 : Saturate  UpperLimit=1.047*5  LowerLimit=-0.5*5
  Saturation9 : Saturate  UpperLimit=1.047*5  LowerLimit=-0.5*5
  Scope : Scope
  Scope27 : Scope
  Sum4 : Sum  Inputs=|+-
  eq2 : Mux  Inputs=3
  angular acc : Outport
  wires:
  angular rate feedback/1 -> Sum4/2
  PID Controller9/1 -> Saturation8/1
  Saturation4/1 -> eq2/1
  eq2/1 -> angular acc/1, Scope27/1, Integrator2/1
  PID Controller3/1 -> Saturation9/1
  Integrator2/1 -> Scope/1
  Saturation9/1 -> eq2/3
  Saturation8/1 -> eq2/2
  Demux3/3 -> PID Controller3/1
  rate setpoint/1 -> Sum4/1
  PID Controller12/1 -> Saturation4/1
  Demux3/2 -> PID Controller9/1
  Demux3/1 -> PID Controller12/1
  Sum4/1 -> Demux3/1

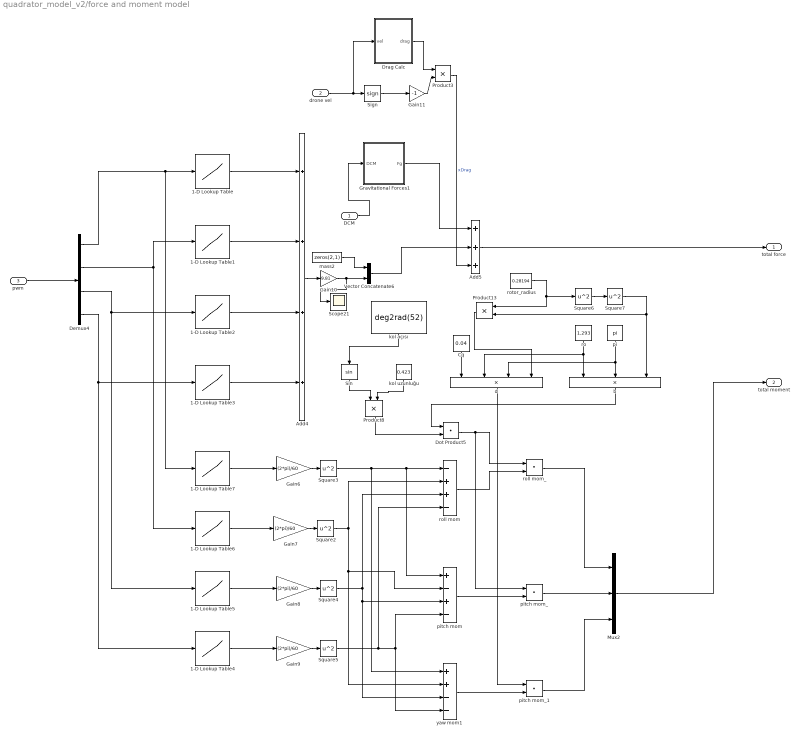
== system quadrator_model_v2/force and moment model ==
  DCM : Inport
  drone vel : Inport  Port=2
  pwm : Inport  Port=3
  1-D Lookup Table{,1..3} (4 alike) : Lookup_n-D  NumberOfTableDimensions=1  BreakpointsForDimension1=l(:,2)  BreakpointsForDimension2=[1000 2000]  Table=l(:,5)  InternalRulePriority=Speed  RndMeth=Simplest
  1-D Lookup Table{4..7} (4 alike) : Lookup_n-D  NumberOfTableDimensions=1  BreakpointsForDimension1=l(:,2)  BreakpointsForDimension2=[1000 2000]  Table=l(:,8)  InternalRulePriority=Speed  RndMeth=Simplest
  Add4 : Sum  Inputs=++++
  Add5 : Sum  Inputs=+++
  Cq : Constant  Value=0.04
  Demux4 : Demux
  Dot Product5 : DotProduct  OutDataTypeStr=Inherit: Inherit via internal rule
  Drag Calc : Subsystem
  Gain10 : Gain  Gain=9.81
  Gain11 : Gain  Gain=-1
  Gain{6..9} (4 alike) : Gain  Gain=(2*pi)/60
  Gravitational Forces1 : Subsystem
  Mux2 : Mux  Inputs=3
  Product13 : Product
  Product3 : Product  RndMeth=Zero
  Product8 : Product
  Scope21 : Scope
  Sign : Signum  ZeroCross=off
  Sin : Trigonometry
  Square{2..7} (6 alike) : Math  Operator=square
  Vector Concatenate6 : Concatenate  ConcatenateDimension=2
  b : Product  Inputs=3
  d : Product  Inputs=4
  kol açısı : Constant  Value=deg2rad(52)
  kol uzunluğu : Constant  Value=0.423
  mass2 : Constant  Value=zeros(2,1)  VectorParams1D=off
  pi : Constant  Value=pi
  pitch mom : Sum  Inputs=+-+-
  pitch mom_ : DotProduct  OutDataTypeStr=Inherit: Inherit via internal rule
  pitch mom_1 : DotProduct  OutDataTypeStr=Inherit: Inherit via internal rule
  ro : Constant  Value=1.293
  roll mom : Sum  Inputs=-++-
  roll mom_ : DotProduct  OutDataTypeStr=Inherit: Inherit via internal rule
  rotor_radius : Constant  Value=0.28194
  yaw mom1 : Sum  Inputs=++--
  total force : Outport
  total moment : Outport  Port=2
  wires:
  Mux2/1 -> total moment/1
  Product3/1 -> Add5/3  "xDrag"
  DCM/1 -> Gravitational Forces1/1(DCM)
  Gain10/1 -> Scope21/1, Vector Concatenate6/2
  Gain7/1 -> Square2/1
  Add4/1 -> Gain10/1
  Square5/1 -> roll mom/4, yaw mom1/4, pitch mom/4
  Sin/1 -> Product8/1
  pwm/1 -> Demux4/1
  Square7/1 -> b/3, Product13/2
  mass2/1 -> Vector Concatenate6/1
  1-D Lookup Table2/1 -> Add4/3
  Product8/1 -> Dot Product5/2
  Gain11/1 -> Product3/2
  Drag Calc/1(drag) -> Product3/1
  pitch mom_1/1 -> Mux2/3
  Square3/1 -> yaw mom1/1, roll mom/1, pitch mom/1
  Square6/1 -> Square7/1
  Square2/1 -> yaw mom1/2, pitch mom/2, roll mom/2
  Cq/1 -> d/1
  kol açısı/1 -> Sin/1
  pitch mom_/1 -> Mux2/2
  yaw mom1/1 -> pitch mom_1/2
  Vector Concatenate6/1 -> Add5/2
  kol uzunluğu/1 -> Product8/2
  1-D Lookup Table3/1 -> Add4/4
  drone vel/1 -> Sign/1, Drag Calc/1(vel)
  1-D Lookup Table5/1 -> Gain8/1
  1-D Lookup Table/1 -> Add4/1
  1-D Lookup Table1/1 -> Add4/2
  Demux4/2 -> 1-D Lookup Table6/1, 1-D Lookup Table1/1
  Square4/1 -> pitch mom/3, yaw mom1/3, roll mom/3
  ro/1 -> b/1, d/2
  1-D Lookup Table4/1 -> Gain9/1
  rotor_radius/1 -> Square6/1, Product13/1
  Gain8/1 -> Square4/1
  Dot Product5/1 -> pitch mom_/1, roll mom_/1
  Demux4/1 -> 1-D Lookup Table7/1, 1-D Lookup Table/1
  Product13/1 -> d/4
  Gravitational Forces1/1(Fg) -> Add5/1
  1-D Lookup Table6/1 -> Gain7/1
  1-D Lookup Table7/1 -> Gain6/1
  Sign/1 -> Gain11/1
  roll mom/1 -> roll mom_/2
  roll mom_/1 -> Mux2/1
  Demux4/4 -> 1-D Lookup Table3/1, 1-D Lookup Table4/1
  pi/1 -> b/2, d/3
  Add5/1 -> total force/1
  pitch mom/1 -> pitch mom_/2
  Demux4/3 -> 1-D Lookup Table2/1, 1-D Lookup Table5/1
  b/1 -> Dot Product5/1
  Gain9/1 -> Square5/1
  Gain6/1 -> Square3/1
  d/1 -> pitch mom_1/1

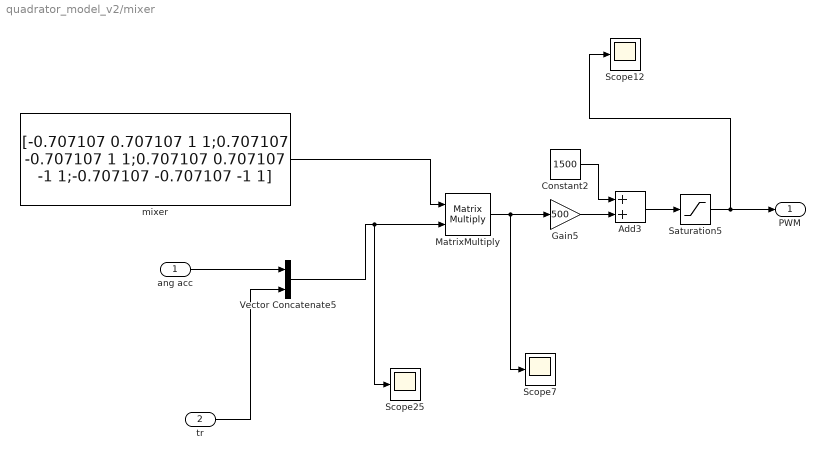
== system quadrator_model_v2/mixer ==
  ang acc : Inport
  tr : Inport  Port=2
  Add3 : Sum
  Constant2 : Constant  Value=1500
  Gain5 : Gain  Gain=500
  MatrixMultiply : Product  Multiplication=Matrix(*)
  Saturation5 : Saturate  UpperLimit=2000  LowerLimit=1000
  Scope12 : Scope
  Scope25 : Scope
  Scope7 : Scope
  Vector Concatenate5 : Concatenate
  mixer : Constant  Value=[-0.707107 0.707107 1 1;0.707107 -0.707107 1 1;0.707107 0.707107 -1 1;-0.707107 -0.707107 -1 1]
  PWM : Outport
  wires:
  mixer/1 -> MatrixMultiply/1
  Add3/1 -> Saturation5/1
  Gain5/1 -> Add3/2
  Constant2/1 -> Add3/1
  ang acc/1 -> Vector Concatenate5/1
  Vector Concatenate5/1 -> MatrixMultiply/2, Scope25/1
  MatrixMultiply/1 -> Gain5/1, Scope7/1
  tr/1 -> Vector Concatenate5/2
  Saturation5/1 -> PWM/1, Scope12/1
